simulink model "lookup_nD_TestGen30"  (R2017b)
settings: Solver=FixedStepDiscrete  StartTime=0.0  StopTime=10.0  RelTol=1e-3
model workspace (MAT data in the model file):
  LUTObjLKnD30 = Simulink.LookupTable
  LUTObjLKnD30.Table = Simulink.lookuptable.Table
  LUTObjLKnD30.Table.Value = reshape([4 16 10 4 16 10 4 16 10 4 16 10 4 16 10 4 16 10 5 19 18 5 19 18 5 19 18 5 19 18 5 19 18 5 19 18 6 20 23 6 20 23 6 20 23 6 20 23 6 20 23 6 20 23 7 21 24 7 21 24 7 21 24 7 21 24 7 21 24 7 21 24 8 22 25 8 22 25 8 22 25 8 22 25 8 22 25 8 22 25 4 16 10 4 16 10 4 16 10 4 16 10 4 16 10 4 16 10 5 19 18 5 19 18 5 19 18 5 19 18 5 19 18 5 19 18 6 20 23 6 20 23 6 20 23 6 20 23 6 20 23 6 20 23 7 21 24 7 21 24 7 21 24 7 21 24 7 21 24 7 21 24 8 22 25 8 22 25 8 22 25 8 22 25 8 22 25 8 22 25], [2 5 3 2 3])
  LUTObjLKnD30.Table.Dimensions = [2 5 3 2 3]
  LUTObjLKnD30.Table.DataType = 'auto'
  LUTObjLKnD30.Table.FieldName = 'Table'
  LUTObjLKnD30.BreakpointsSpecification = 'Even spacing'
  LUTObjLKnD30.Breakpoints(1) = Simulink.lookuptable.Evenspacing
  LUTObjLKnD30.Breakpoints(1).FirstPoint = 23.7419515717
  LUTObjLKnD30.Breakpoints(1).Spacing = 1.5
  LUTObjLKnD30.Breakpoints(1).FirstPointName = 'BPFirstPoint1'
  LUTObjLKnD30.Breakpoints(1).SpacingName = 'BPSpacing1'
  LUTObjLKnD30.Breakpoints(1).TunableSizeName = 'N1'
  LUTObjLKnD30.Breakpoints(1).DataType = 'auto'
  LUTObjLKnD30.Breakpoints(1).FieldName = 'BP1'
  LUTObjLKnD30.Breakpoints(2) = Simulink.lookuptable.Evenspacing
  LUTObjLKnD30.Breakpoints(2).FirstPoint = 10.0835203458
  LUTObjLKnD30.Breakpoints(2).Spacing = 1.5
  LUTObjLKnD30.Breakpoints(2).FirstPointName = 'BPFirstPoint2'
  LUTObjLKnD30.Breakpoints(2).SpacingName = 'BPSpacing2'
  LUTObjLKnD30.Breakpoints(2).TunableSizeName = 'N2'
  LUTObjLKnD30.Breakpoints(2).DataType = 'auto'
  LUTObjLKnD30.Breakpoints(2).FieldName = 'BP2'
  LUTObjLKnD30.Breakpoints(3) = Simulink.lookuptable.Evenspacing
  LUTObjLKnD30.Breakpoints(3).FirstPoint = 11.5526886261
  LUTObjLKnD30.Breakpoints(3).Spacing = 1.5
  LUTObjLKnD30.Breakpoints(3).FirstPointName = 'BPFirstPoint3'
  LUTObjLKnD30.Breakpoints(3).SpacingName = 'BPSpacing3'
  LUTObjLKnD30.Breakpoints(3).TunableSizeName = 'N3'
  LUTObjLKnD30.Breakpoints(3).DataType = 'auto'
  LUTObjLKnD30.Breakpoints(3).FieldName = 'BP3'
  LUTObjLKnD30.Breakpoints(4) = Simulink.lookuptable.Evenspacing
  LUTObjLKnD30.Breakpoints(4).FirstPoint = 95.8229442383
  LUTObjLKnD30.Breakpoints(4).Spacing = 1.5
  LUTObjLKnD30.Breakpoints(4).FirstPointName = 'BPFirstPoint4'
  LUTObjLKnD30.Breakpoints(4).SpacingName = 'BPSpacing4'
  LUTObjLKnD30.Breakpoints(4).TunableSizeName = 'N4'
  LUTObjLKnD30.Breakpoints(4).DataType = 'auto'
  LUTObjLKnD30.Breakpoints(4).FieldName = 'BP4'
  LUTObjLKnD30.Breakpoints(5) = Simulink.lookuptable.Evenspacing
  LUTObjLKnD30.Breakpoints(5).FirstPoint = 117.445774373
  LUTObjLKnD30.Breakpoints(5).Spacing = 1.5
  LUTObjLKnD30.Breakpoints(5).FirstPointName = 'BPFirstPoint5'
  LUTObjLKnD30.Breakpoints(5).SpacingName = 'BPSpacing5'
  LUTObjLKnD30.Breakpoints(5).TunableSizeName = 'N5'
  LUTObjLKnD30.Breakpoints(5).DataType = 'auto'
  LUTObjLKnD30.Breakpoints(5).FieldName = 'BP5'
  LUTObjLKnD30.SupportTunableSize = 0
  LUTObjLKnD30.StructTypeInfo = Simulink.lookuptable.StructTypeInfo
  LUTObjLKnD30.StructTypeInfo.Name = 'LUT'
  LUTObjLKnD30.StructTypeInfo.DataScope = 'Auto'
settings Model: Creator=ktrinh  LastModifiedBy=ktrinh
settings DebuggingCC: ParameterOverflowMsg=none

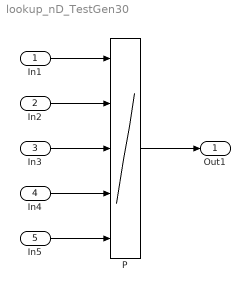
== system lookup_nD_TestGen30 ==
  In1 : Inport  OutMin=0  OutMax=127  PortDimensions=1
  In2 : Inport  Port=2  OutMin=0  OutMax=127
  In3 : Inport  Port=3  OutMin=0  OutMax=127
  In4 : Inport  Port=4  OutMin=0  OutMax=127
  In5 : Inport  Port=5  OutMin=0  OutMax=127
  P : Lookup_n-D  NumberOfTableDimensions=5  DataSpecification=Lookup table object  LookupTableObject=LUTObjLKnD30  BreakpointsSpecification=Even spacing  BreakpointsForDimension3=[5, 7]  Table=reshape(repmat([4 5 6;16 19 20;10 18 23],1,2),[3,3,2])  InternalRulePriority=Speed  RndMeth=Simplest  InputSameDT=on
  Out1 : Outport
  wires:
  In1/1 -> P/1
  In2/1 -> P/2
  In3/1 -> P/3
  In4/1 -> P/4
  In5/1 -> P/5
  P/1 -> Out1/1
